simulink model "Lab_5_Part_B"  (R2021a)
settings: Solver=VariableStepAuto  StartTime=0.0  StopTime=5  RelTol=1e-3
settings Model: Creator=ta5996u  LastModifiedBy=ta5996u

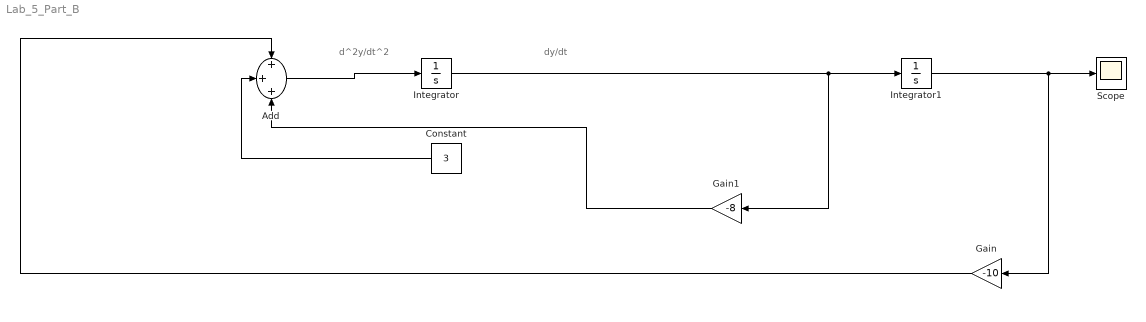
== system Lab_5_Part_B ==
  note: d^2y/dt^2
  note: dy/dt
  Add : Sum  Inputs=+++
  Constant : Constant  Value=3
  Gain : Gain  Gain=-10
  Gain1 : Gain  Gain=-8
  Integrator : Integrator
  Integrator1 : Integrator
  Scope : Scope
  wires:
  Integrator/1 -> Gain1/1, Integrator1/1
  Gain1/1 -> Add/3
  Integrator1/1 -> Gain/1, Scope/1
  Add/1 -> Integrator/1
  Gain/1 -> Add/1
  Constant/1 -> Add/2
